simulink model "bikesim_magic_formula"  (R2026a)
settings: Solver=ode45  MaxStep=1E-03
InitFcn:
  | moto_init;
values from neighbouring files (symbols this model uses):
  p = motoParameters    [bikeSimToMotoParameters.m]    (also in moto_init.m = bikeSimToPrydeV2Parameters(bs,130/3.6); moto_trim_test.m = P{idx_vx}; steadyTurningTrimEqns.m = in3(41,:); steadyTurningTrimJac.m = in3(41,:))
  pr = table2struct(rt.Pacejka)    [moto_init.m]    (also in moto_trim_test.m = fpacejka(bs.RearTire.Pacejka))
libraries: simulink x2, simulink_extras x1
(part 2 of 2)

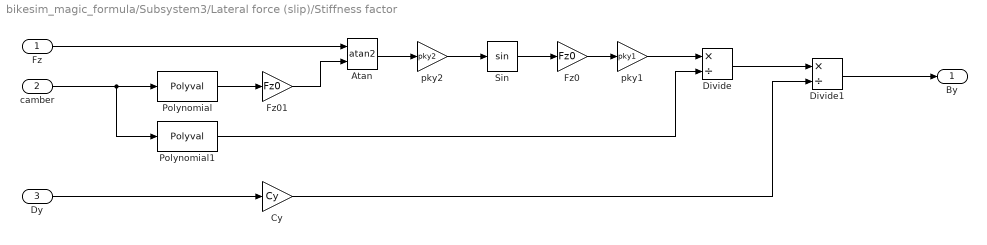
== system bikesim_magic_formula/Subsystem3/Lateral force (slip)/Stiffness factor ==
  Fz : Inport
  camber : Inport  Port=2
  Dy : Inport  Port=3
  Atan : Trigonometry  Operator=atan2
  Cy : Gain  Gain=Cy
  Divide : Product  Inputs=*/
  Divide1 : Product  Inputs=*/
  Fz0 : Gain  Gain=Fz0
  Fz01 : Gain  Gain=Fz0
  Polynomial : Polyval  Coefs=[pky4,0,pky3]
  Polynomial1 : Polyval  Coefs=[pky5,0,1]
  Sin : Trigonometry
  pky1 : Gain  Gain=pky1
  pky2 : Gain  Gain=pky2
  By : Outport
  wires:
  Dy/1 -> Cy/1
  Fz0/1 -> pky1/1
  Sin/1 -> Fz0/1
  pky2/1 -> Sin/1
  Atan/1 -> pky2/1
  Fz/1 -> Atan/1
  Fz01/1 -> Atan/2
  Polynomial/1 -> Fz01/1
  camber/1 -> Polynomial1/1, Polynomial/1
  pky1/1 -> Divide/1
  Polynomial1/1 -> Divide/2
  Divide/1 -> Divide1/1
  Cy/1 -> Divide1/2
  Divide1/1 -> By/1
